simulink model "Sim_2025_04_07_Heet"  (R2024b)
settings: Solver=FixedStepAuto  StartTime=0.0  StopTime=2350  FixedStep=0.01  RelTol=1e-3
values from neighbouring files (symbols this model uses):
  cpSn = 230    [Sim_Parameter_Heet.m]
  mB = VB*rohSn    (= 7671.14496)    [Sim_Parameter_Heet.m]
  TU = 35    [Sim_Parameter_Heet.m]
undefined symbols (not defined in the file or in its folder): PLC_1, SIMATIC, UA
libraries: simulink x7, slpidlib x7, opcualib x6
(part 1 of 3)
settings Model: Creator=hartmann  LastModifiedBy=khamar

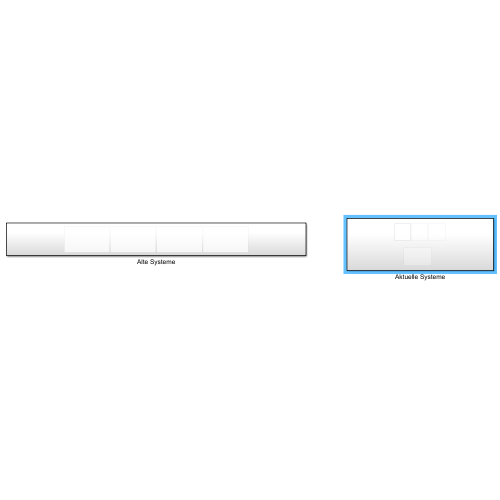
[thumbnail: Simulink's stored preview of the top-level diagram]
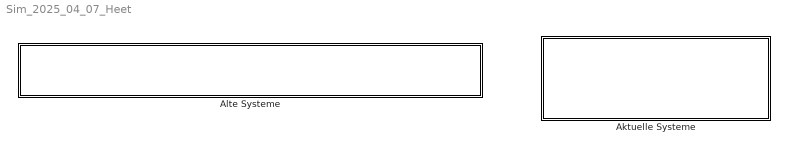
== system Sim_2025_04_07_Heet ==
  Aktuelle Systeme : Subsystem
  Alte Systeme : Subsystem

== system Sim_2025_04_07_Heet/Aktuelle Systeme ==
  Subsystem : Subsystem  Commented=on
  System für Stillstand für Siemens : Subsystem  Commented=on
  System mit Echtdatensätze : Subsystem
  System ohne Echtdatensätze : Subsystem  Commented=on

== system Sim_2025_04_07_Heet/Alte Systeme ==
  Subsystem1 : Subsystem  Commented=on
  Subsystem2 : Subsystem  Commented=on
  Subsystem3 : Subsystem  Commented=on
  Subsystem4 : Subsystem  Commented=on

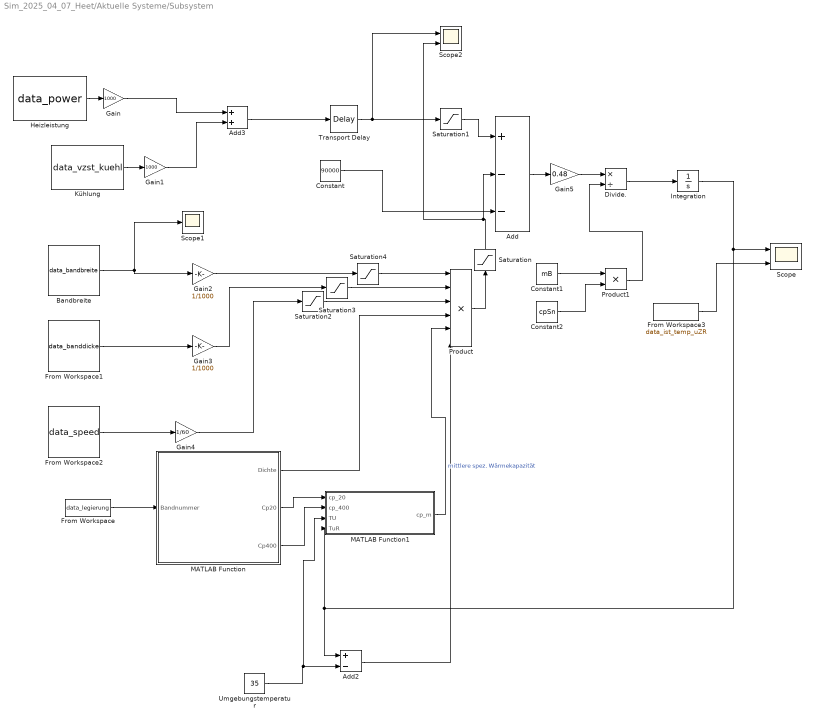
== system Sim_2025_04_07_Heet/Aktuelle Systeme/Subsystem ==
  Add : Sum  Inputs=+--
  Add2 : Sum  Inputs=+-
  Add3 : Sum
  Bandbreite : FromWorkspace  VariableName=data_bandbreite
  Constant : Constant  Value=90000
  Constant1 : Constant  Value=mB
  Constant2 : Constant  Value=cpSn
  Divide. : Product  Inputs=*/
  From Workspace : FromWorkspace  VariableName=data_legierung
  From Workspace1 : FromWorkspace  VariableName=data_banddicke
  From Workspace2 : FromWorkspace  VariableName=data_speed
  From Workspace3 : FromWorkspace  VariableName=data_ist_temp_uZR
  Gain : Gain  Gain=1000
  Gain1 : Gain  Gain=1000
  Gain2 : Gain  Gain=1/1000
  Gain3 : Gain  Gain=1/1000
  Gain4 : Gain  Gain=1/60
  Gain5 : Gain  Gain=0.48
  Heizleistung : FromWorkspace  VariableName=data_power
  Integration : Integrator  InitialCondition=273  IgnoreLimit=on
  Kühlung : FromWorkspace  VariableName=data_vzst_kuehl
  MATLAB Function : MATLAB Function  TreatAsAtomicUnit=on
  MATLAB Function1 : MATLAB Function  TreatAsAtomicUnit=on
  Product : Product  Inputs=6
  Product1 : Product
  Saturation{,1..4} (5 alike) : Saturate  UpperLimit=inf  LowerLimit=0
  Scope : Scope  NumInputPorts=2
  Scope1 : Scope
  Scope2 : Scope  NumInputPorts=2
  Transport Delay : TransportDelay  DelayTime=95
  Umgebungstemperatur : Constant  Value=35
  wires:
  Heizleistung/1 -> Gain/1
  Kühlung/1 -> Gain1/1
  Add3/1 -> Transport Delay/1
  Bandbreite/1 -> Scope1/1, Gain2/1
  From Workspace1/1 -> Gain3/1
  From Workspace2/1 -> Gain4/1
  Product/1 -> Saturation/1
  Divide./1 -> Integration/1
  Integration/1 -> Add2/1, MATLAB Function1/4(TuR), Scope/1
  Add/1 -> Gain5/1
  From Workspace/1 -> MATLAB Function/1(Bandnummer)
  MATLAB Function/1(Dichte) -> Product/4
  MATLAB Function/2(Cp20) -> MATLAB Function1/1(cp_20)
  MATLAB Function/3(Cp400) -> MATLAB Function1/2(cp_400)
  Constant1/1 -> Product1/1
  Constant2/1 -> Product1/2
  Product1/1 -> Divide./2
  Umgebungstemperatur/1 -> MATLAB Function1/3(TU), Add2/2
  Add2/1 -> Product/6
  From Workspace3/1 -> Scope/2
  Saturation/1 -> Scope2/2, Add/2
  Saturation1/1 -> Add/1
  Gain/1 -> Add3/1
  Gain1/1 -> Add3/2
  Gain2/1 -> Saturation4/1
  Gain3/1 -> Saturation3/1
  Gain4/1 -> Saturation2/1
  MATLAB Function1/1(cp_m) -> Product/5  "mittlere spez. Wärmekapazität"
  Constant/1 -> Add/3
  Saturation2/1 -> Product/3
  Saturation3/1 -> Product/2
  Saturation4/1 -> Product/1
  Gain5/1 -> Divide./1
  Transport Delay/1 -> Scope2/1, Saturation1/1

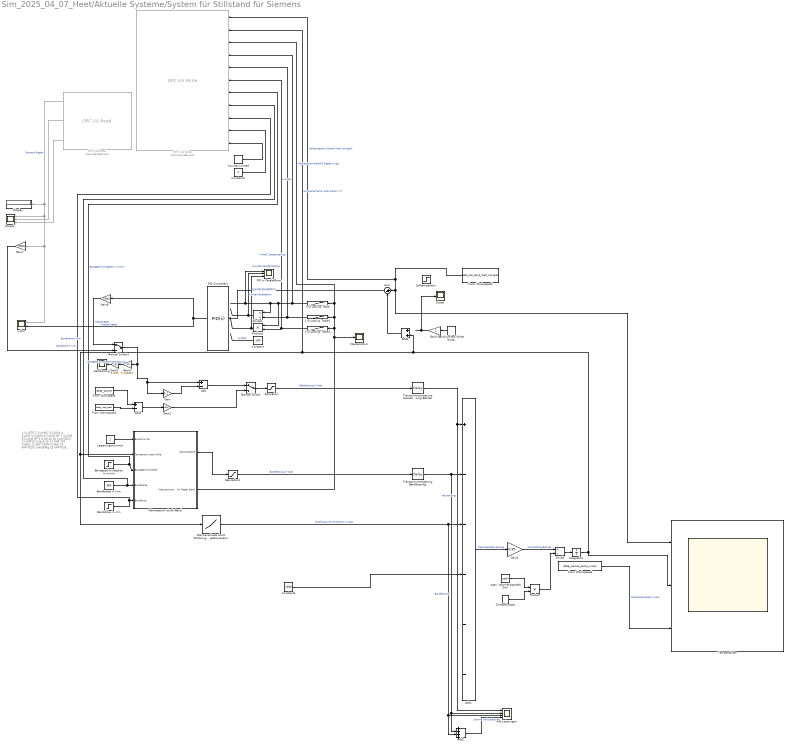
== system Sim_2025_04_07_Heet/Aktuelle Systeme/System für Stillstand für Siemens ==
  note: 1
      | Cu-ETP
      |
      | 2
      | Cu-PHC
      |
      | 3
      | CuSn4
      |
      | 4
      | CuSn5
      |
      | 5
      | CuSn6
      |
      | 6
      | CuSn6 HP
      |
      | 7
      | CuSn8
      |
      | 8
      | CuSn8 HP
      |
      | 9
      | CuSn10
      |
      | 10
      | CuSn3Zn9
      |
      | 11
      | KHP15 CuSn0,15
      |
      | 12
      | KHP 102 CuNiSi
      |
      | 13
      | KHP 102M CuNiSi
      |
      | 14
      | KHP7025 CuNi3SiMg
      |
      | 15
      | KHP7026 CuNi2Si
      |
      | 16
      | KHP105 CuNi1Sn0,5
      |
      | 17
      | KHP109 CuNi1Sn0,9
      |
      | 18
      | C688 CuZn23Al3,5Co
  1-D Lookup Table : Lookup_n-D  NumberOfTableDimensions=1  BreakpointsForDimension1=[0 0.10000000000000001 0.20000000000000001 0.29999999999999999 0.40000000000000002 0.5 0.59999999999999998 0.69999999999999996 0.80000000000000004 0.90000000000000002 1 1.1000000000000001 1.2 1.3 1.3999999999999999 1.5 1.6000000000000001 1.7 1.8 1.8999999999999999 2 2.1000000000000001 2.2000000000000002 2.2999999999999998 2.3999999999999999 2.5 2.6000000000000001 2.7000000000000002 2.7999999999999998 2.8999999999999999 3 3.1000000000000001 3.2000000000000002 3.2999999999999998 3.3999999999999999 3.5 3.6000000000000001 3.7000000000000002 3.7999999999999998 3.8999999999999999 4 4.0999999999999996 4.2000000000000002 4.2999999999999998 4.4000000000000004 4.5]  Table=[5;5.07;5.13;5.2;5.27;5.33;5.4;5.47;5.53;5.6;5.67;5.73;5.8;5.87;5.93;6;6.07;6.13;6.2;6.27;6.33;6.4;6.47;6.53;6.6;6.67;6.73;6.8;6.87;6.93;7;7.07;7.13;7.2;7.27;7.33;7.4;7.47;7.53;7.6;7.67;7.73;7.8;7.87;7.93;8]  InternalRulePriority=Speed  RndMeth=Simplest
  1-D Lookup Table1 : Lookup_n-D  NumberOfTableDimensions=1  BreakpointsForDimension1=[0 0.10000000000000001 0.20000000000000001 0.29999999999999999 0.40000000000000002 0.5 0.59999999999999998 0.69999999999999996 0.80000000000000004 0.90000000000000002 1 1.1000000000000001 1.2 1.3 1.3999999999999999 1.5 1.6000000000000001 1.7 1.8 1.8999999999999999 2 2.1000000000000001 2.2000000000000002 2.2999999999999998 2.3999999999999999 2.5 2.6000000000000001 2.7000000000000002 2.7999999999999998 2.8999999999999999 3 3.1000000000000001 3.2000000000000002 3.2999999999999998 3.3999999999999999 3.5 3.6000000000000001 3.7000000000000002 3.7999999999999998 3.8999999999999999 4 4.0999999999999996 4.2000000000000002 4.2999999999999998 4.4000000000000004 4.5]  Table=[285.7;253.3;256.7;260;263.3;266.7;270;273.3;276.7;280;283.3;286.7;290;293.3;296.7;300;303.3;306.7;310;313.3;316.7;320;323.3;326.7;330;333.3;336.7;340;343.3;346.7;350;353.3;356.7;360;363.3;366.7;370;373.3;376.7;380;383.3;386.7;390;393.3;396.7;400]  InternalRulePriority=Speed  RndMeth=Simplest
  1-D Lookup Table2 : Lookup_n-D  NumberOfTableDimensions=1  BreakpointsForDimension1=[0 0.10000000000000001 0.20000000000000001 0.29999999999999999 0.40000000000000002 0.5 0.59999999999999998 0.69999999999999996 0.80000000000000004 0.90000000000000002 1 1.1000000000000001 1.2 1.3 1.3999999999999999 1.5 1.6000000000000001 1.7 1.8 1.8999999999999999 2 2.1000000000000001 2.2000000000000002 2.2999999999999998 2.3999999999999999 2.5 2.6000000000000001 2.7000000000000002 2.7999999999999998 2.8999999999999999 3 3.1000000000000001 3.2000000000000002 3.2999999999999998 3.3999999999999999 3.5 3.6000000000000001 3.7000000000000002 3.7999999999999998 3.8999999999999999 4 4.0999999999999996 4.2000000000000002 4.2999999999999998 4.4000000000000004 4.5]  Table=[8;59.2;58.4;57.7;57;56.3;55.6;54.9;54.2;53.6;52.9;52.3;51.7;51.1;50.6;50;49.5;48.9;48.4;47.9;47.4;46.9;46.4;45.9;45.5;45;44.6;44.1;43.7;43.3;42.9;42.5;42.1;41.7;41.3;40.9;40.5;40.2;39.8;39.5;39.1;38.8;38.5;38.1;37.8;37.5]  InternalRulePriority=Speed  RndMeth=Simplest
  Add : Sum  Inputs=+-
  Add1 : Sum  Inputs=+-----
  Add2 : Sum  Inputs=++++
  Add3 : Sum
  Add4 : Sum  Inputs=+-
  Alle Leistungen : Scope  NumInputPorts=6
  Band-Limited White Noise : simulink/Sources/Band-Limited White Noise  Cov=[0.1]  Ts=20  seed=[23341]
  Bandbreite in mm : Constant  Value=360
  Banddicke in mm : Step  Time=3000  Before=0.15  After=0.5  SampleTime=0
  Bandgeschwindigkeit in m/min : Step  Time=2000  After=0  SampleTime=0
  Constant : Constant  Value=100
  Constant1 : Constant  Value=-1000
  Constant2 : Constant
  Counter Limited : simulink/Sources/Counter Limited  uplimit=100  tsamp=-1
  Display : Display
  Divide : Product  Inputs=*/
  Divide1 : Product  Inputs=*/
  From Workspace : FromWorkspace  VariableName=data_power
  From Workspace1 : FromWorkspace  VariableName=data_vzst_kuehl
  From Workspace2 : FromWorkspace  VariableName=data_soll_temp_start_korrigiert
  From Workspace3 : FromWorkspace  VariableName=data_wanne_temp_innen
  Gain : Gain  Gain=0.1
  Gain1 : Gain
  Gain2 : Gain  Gain=1000
  Gain3 : Gain  Gain=0.95
  Gain4 : Gain  Gain=0.142857
  Gain5 : Gain  Gain=0.001
  Gain7 : Gain  Gain=7000
  Gain9 : Gain  Gain=7000
  Heizleistung : Scope
  Integration : Integrator  InitialCondition=276.5  IgnoreLimit=on
  Legierungsnummer : Constant
  Manual Switch : ManualSwitch
  Manual Switch1 : ManualSwitch
  Massenstrom : Scope
  OPC UA Read : opcualib/OPC UA Read  Commented=on  SelectedServer=SIMATIC.S7-1500.OPC-UA.Application:PLC_1  ServerList=SIMATIC.S7-1500.OPC-UA.Application:PLC_1  NodeList={ '1', 'reStellwert', '4', '2', '1' }  ShowQualityPort=on  ShowTimestampPort=on  ShowTimestampPortAs=Seconds since start  SampleTime=-1
  OPC UA Write : opcualib/OPC UA Write  Commented=on  SelectedServer=SIMATIC.S7-1500.OPC-UA.Application:PLC_1  ServerList=SIMATIC.S7-1500.OPC-UA.Application:PLC_1  SampleTime=-1  NodeList={ '1', 'reSollwert', '4', '3', '1'; '2', 'reIstTemperaturVonStreckensimulation', '4', '4', '1'; '3', 'reMassenfluss', '4', '5', '1'; '4', 'reP_Anteil', '4', '6', '1'; '5', 'reI_Anteil', '4', '7', '1'; '6', 'reD_Anteil', '4', '8', '1'; '7', 'reGeschwindigkeit', '4', '9', '1'; '8', 'reBandbreite', '4', '10', '1'; '9', 'reBanddicke', '4', '11', '1'; '10', 'boRunVonSimulink', '4', '12', '1'; '11', 'iLifeRegister', '4', '13', '1' }
  PID Controller1 : slpidlib/PID Controller  Controller=PID  Form=Parallel  TimeDomain=Continuous-time  UseExternalTs=off  SampleTime=-1  IntegratorMethod=Forward Euler  FilterMethod=Forward Euler  ControllerParametersSource=internal  P=5  I=0.0175  UseKiTs=off  D=40  UseExternalDerivativeSource=off  N=1  UseFilter=on  TunerSelectOption=Transfer Function Based (PID Tuner App)  InitialConditionSource=internal  InitialConditionForIntegrator=0  InitialConditionForFilter=0  DifferentiatorICPrevScaledInput=0  ExternalReset=none  TrackingMode=off  Kt=1  LimitOutput=on  SatLimitsSource=internal  UpperSaturationLimit=100  LowerSaturationLimit=0  LinearizeAsGain=on  AntiWindupMode=none  Kb=1  LimitIntegrator=off  UpperIntegratorSaturationLimit=inf  LowerIntegratorSaturationLimit=-inf  POutMin=[]  POutMax=[]  IOutMin=[]  IOutMax=[]  DOutMin=[]  DOutMax=[]  NOutMin=[]  NOutMax=[]  SumOutMin=[]  SumOutMax=[]  SaturationOutMin=[]  SaturationOutMax=[]  PParamMin=[]  PParamMax=[]  IParamMin=[]  IParamMax=[]  DParamMin=[]  DParamMax=[]  NParamMin=[]  NParamMax=[]  KbParamMin=[]  KbParamMax=[]  KtParamMin=[]  KtParamMax=[]  KbOutMin=[]  KbOutMax=[]  KtOutMin=[]  KtOutMax=[]  IntegratorOutMin=[]  IntegratorOutMax=[]  FilterOutMin=[]  FilterOutMax=[]  SumI1OutMin=[]  SumI1OutMax=[]  SumI2OutMin=[]  SumI2OutMax=[]  SumI3OutMin=[]  SumI3OutMax=[]  SumI4OutMin=[]  SumI4OutMax=[]  SumDOutMin=[]  SumDOutMax=[]  DifferentiatorOutMin=[]  DifferentiatorOutMax=[]  FilterDiffOutCoefMin=[]  FilterDiffOutCoefMax=[]  ReciprocalOutMin=[]  ReciprocalOutMax=[]  SumDenOutMin=[]  SumDenOutMax=[]  SumNumOutMin=[]  SumNumOutMax=[]  DivideOutMin=[]  DivideOutMax=[]  UdiffTsProdOutMin=[]  UdiffTsProdOutMax=[]  NTsProdOutMin=[]  NTsProdOutMax=[]  UintegralTsProdOutMin=[]  UintegralTsProdOutMax=[]  UngainTsProdOutMin=[]  UngainTsProdOutMax=[]  ClampingZeroOutDataTypeStr=Inherit: Inherit via back propagation  ClampingZeroOutMin=[]  ClampingZeroOutMax=[]  FilterDenConstantOutDataTypeStr=Inherit: Inherit via back propagation  FilterDenConstantOutMin=[]  FilterDenConstantOutMax=[]  PCopyOutDataTypeStr=Inherit: Inherit via back propagation  PCopyOutMin=[]  PCopyOutMax=[]  NCopyOutDataTypeStr=Inherit: Inherit via back propagation  NCopyOutMin=[]  NCopyOutMax=[]  IntegratorContinuousStateAttributes=''  IntegratorStateMustResolveToSignalObject=off  IntegratorRTWStateStorageClass=Auto  FilterContinuousStateAttributes=''  FilterStateMustResolveToSignalObject=off  FilterRTWStateStorageClass=Auto  ParallelPVariant=InternalParameters  IdealPVariant=Disabled  IVariant=InternalParameters  DVariant=InternalParameters  IntegratorVariant=Continuous  SatVariant=Enabled  AWVariant=Passthrough  PCopyVariant=Disabled  TRVariant=Disabled  FdbkBlocksVariant=Forward  IdealPFdbkVariant=Disabled  SatFdbkVariant=Disabled  DerivativeFilterVariant=ContFilter  NVariant=InternalParameters  NCopyVariant=Disabled  FilterICVariant=InternalICsFilter  IntegratorICVariant=InternalICs  ExternalResetVariant=Disabled  TRSumVariant=Passthrough  SumFdbkVariant=Disabled  SumVariant=Sum_PID  TsampFilterVariant=InternalTs  TsampNgainVariant=Passthrough  TsampIntegralVariant=Disabled_SignalSpec  ExternalSaturationOutDataTypeStr=Inherit: Same as second input  DerivativeSourceVariant=ErrorSignal  PreIntVariant=InternalPreInt
  PID in Paralellform : Scope  NumInputPorts=3
  Product : Product
  Product1 : Product
  Saturation : Saturate  UpperLimit=inf  LowerLimit=0
  Saturation1 : Saturate  UpperLimit=inf  LowerLimit=0
  Scope : Scope
  Scope1 : Scope  NumInputPorts=3
  Solltemperatur : Step  Time=1000  Before=277  After=279  SampleTime=0
  Sum : Sum  Inputs=|+-
  Temperaturen : Scope  NumInputPorts=3
  Transportverzögerung Bandleistung : TransportDelay  DelayTime=5
  Transportverzögerung Heizleistung Betrieb : TransportDelay  DelayTime=63  BufferSize=15000
  Wärmestrom durch Band : Subsystem
  "Wärmeverluste durch Strahlung und Konvektion in Abhängigkeit der Zinntemperatur, mit fester Umgebungstemperatur" : Lookup_n-D  NumberOfTableDimensions=1  BreakpointsForDimension1=[0 250 260 270 280 290 300 310 320]  Table=[0;15000;15200;15400;15600;15800;16000;16200;16400]  InternalRulePriority=Speed  RndMeth=Simplest
  Zinnbadmasse : Constant  Value=7700
  spez. Wärmekapazität Zinn : Constant  Value=cpSn
  y-Out : Scope  NumInputPorts=2
  wires:
  Product/1 -> Divide/2
  Saturation1/1 -> Transportverzögerung Bandleistung/1  "Bandleistung in Watt"
  PID Controller1/1 -> Gain9/1, y-Out/2  "Matlab-Regler"
  Transportverzögerung Bandleistung/1 -> Alle Leistungen/3, Add2/2, Add1/2  "Bandleistung"
  Banddicke in mm/1 -> OPC UA Write/9, Wärmestrom durch Band/5(Banddicke)  "Banddicke in mm"
  Legierungsnummer/1 -> Wärmestrom durch Band/1(Bandnummer)
  Saturation/1 -> Transportverzögerung Heizleistung Betrieb/1  "Ofenleistung in Watt"
  Gain5/1 -> Heizleistung/1  "Geregelte simulierte Heizleistung"
  Bandgeschwindigkeit in m/min/1 -> OPC UA Write/7, Wärmestrom durch Band/3(Bandgeschwindikeit)  "Bandgeschwindigkeit in m/min"
  Gain4/1 -> Gain5/1
  spez. Wärmekapazität Zinn/1 -> Product/1
  Divide/1 -> Integration/1
  Sum/1 -> PID Controller1/1
  Integration/1 -> OPC UA Write/2, Wärmestrom durch Band/2(Temperatur unter Rolle), "Wärmeverluste durch Strahlung und Konvektion in Abhängigkeit der Zinntemperatur, mit fester Umgebungstemperatur"/1, Add3/2, Temperaturen/2  "Simulierte Temp. unter Rolle in °C"
  Zinnbadmasse/1 -> Product/2
  "Wärmeverluste durch Strahlung und Konvektion in Abhängigkeit der Zinntemperatur, mit fester Umgebungstemperatur"/1 -> Alle Leistungen/4, Add2/3, Add1/3  "Strahlung und Konvektion in Watt"
  Gain3/1 -> Divide/1  "Wirkleistung Betrieb"
  Wärmestrom durch Band/1(Leistung Band) -> Saturation1/1
  Constant/1 -> ?  "N-Filter"
  Wärmestrom durch Band/2(Massenstrom für Regler Band) -> Massenstrom/1, OPC UA Write/3, 1-D Lookup Table/1, 1-D Lookup Table1/1, 1-D Lookup Table2/1  "Massenstrom Band für Regler in kg/s"
  From Workspace2/1 -> OPC UA Write/1, Temperaturen/1, Sum/1  "Solltemperatur Wanne innen korrigiert"
  Transportverzögerung Heizleistung Betrieb/1 -> Alle Leistungen/1, Add1/1  "Heizleistung"
  Add/1 -> Manual Switch/1
  OPC UA Read/2 -> Scope1/2
  OPC UA Read/1 -> Display/1, Scope1/1, Gain7/1, y-Out/1  "Siemens-Regler"
  OPC UA Read/3 -> Scope1/3
  Add2/1 -> Alle Leistungen/6  "Summe Verlustleistung"
  Add1/1 -> Gain3/1  "Resultierende Leistung"
  Constant2/1 -> OPC UA Write/10
  Counter Limited/1 -> OPC UA Write/11
  Gain7/1 -> Manual Switch1/2
  Gain9/1 -> Manual Switch1/1  "Matlabregler"
  1-D Lookup Table/1 -> Product1/1, Divide1/1, PID in Paralellform/1, OPC UA Write/4  "P-Anteil"
  1-D Lookup Table1/1 -> OPC UA Write/5, Divide1/2  "I-Anteil Zeitdarstellung"
  1-D Lookup Table2/1 -> Product1/2, OPC UA Write/6  "D-Anteil Zeitdarstellung"
  Bandbreite in mm/1 -> OPC UA Write/8, Wärmestrom durch Band/4(Bandbreite)  "Bandbreite in mm"
  Divide1/1 -> PID in Paralellform/2  "I-Anteil Parallelform"
  Product1/1 -> PID in Paralellform/3  "D-Anteil Paralellform"
  Gain/1 -> Add/2
  Band-Limited White Noise/1 -> Gain1/1
  Add3/1 -> Sum/2
  Gain1/1 -> Scope/1
  From Workspace/1 -> Add4/1
  Manual Switch1/1 -> Gain/1, Add/1, Gain4/1
  From Workspace1/1 -> Add4/2
  Add4/1 -> Gain2/1
  Manual Switch/1 -> Saturation/1
  Gain2/1 -> Manual Switch/2
  Constant1/1 -> Add1/4
  From Workspace3/1 -> Temperaturen/3  "Wannentemperatur innen"
  ? -> ?  "Temperatur unter Rolle"
  ? -> ?  "Soll-Temp. unter Rolle"
  ? -> ?  "Wannentemperatur außen"
  ? -> ?  "Solltemperatur Wanne innen Rezept"

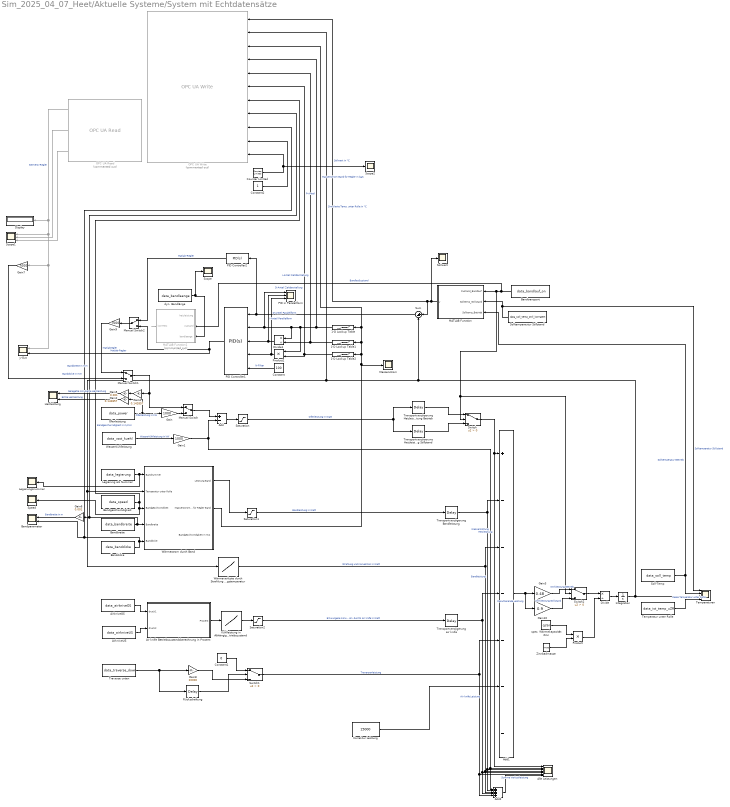
== system Sim_2025_04_07_Heet/Aktuelle Systeme/System mit Echtdatensätze ==
  1-D Lookup Table : Lookup_n-D  NumberOfTableDimensions=1  BreakpointsForDimension1=[0 0.29999999999999999 0.59999999999999998 0.90000000000000002 1.2 1.5 1.8 2.1000000000000001 2.3999999999999999 2.7000000000000002 3 3.2999999999999998 3.6000000000000001 3.8999999999999999 4.2000000000000002 4.5]  Table=[5;5.2;5.4;5.6;5.8;6;6.2;6.4;6.6;6.8;7;7.2;7.4;7.6;7.8;8]  InternalRulePriority=Speed  RndMeth=Simplest
  1-D Lookup Table1 : Lookup_n-D  NumberOfTableDimensions=1  BreakpointsForDimension1=[0 0.29999999999999999 0.59999999999999998 0.90000000000000002 1.2 1.5 1.8 2.1000000000000001 2.3999999999999999 2.7000000000000002 3 3.2999999999999998 3.6000000000000001 3.8999999999999999 4.2000000000000002 4.5]  Table=[250;260;270;280;290;300;310;320;330;340;350;360;370;380;390;400]  InternalRulePriority=Speed  RndMeth=Simplest
  1-D Lookup Table2 : Lookup_n-D  NumberOfTableDimensions=1  BreakpointsForDimension1=[0 0.29999999999999999 0.59999999999999998 0.90000000000000002 1.2 1.5 1.8 2.1000000000000001 2.3999999999999999 2.7000000000000002 3 3.2999999999999998 3.6000000000000001 3.8999999999999999 4.2000000000000002 4.5]  Table=[60;57.7;55.6;53.6;51.7;50;48.4;46.9;45.5;44.1;42.9;41.7;40.5;39.5;38.5;37.5]  InternalRulePriority=Speed  RndMeth=Simplest
  Add : Sum  Inputs=+-
  Add1 : Sum  Inputs=+------
  Add2 : Sum  Inputs=+++++
  Air knife Betriebszustandsberechnung in Prozent : MATLAB Function  TreatAsAtomicUnit=on  SystemSampleTime=0.1
  AirkniveOS : FromWorkspace  VariableName=data_airkniveOS  SampleTime=-1
  AirkniveUS : FromWorkspace  VariableName=data_airkniveUS  SampleTime=-1
  Alle Leistungen : Scope  NumInputPorts=7
  Bandbreite : FromWorkspace  VariableName=data_bandbreite  SampleTime=-1
  Banddicke : FromWorkspace  VariableName=data_banddicke  SampleTime=-1
  Bandgeschwindigkeit : FromWorkspace  VariableName=data_speed  SampleTime=-1
  Bandparameter : Scope  NumInputPorts=2
  Bandtransport : FromWorkspace  VariableName=data_bandlauf_on  SampleTime=-1
  Constant : Constant  Value=100
  Constant1 : Constant  Value=0
  Constant2 : Constant
  Counter Limited : simulink/Sources/Counter Limited  uplimit=100  tsamp=-1
  Display : Display
  Divide : Product  Inputs=*/
  Divide1 : Product  Inputs=*/  OutMin=[eps]
  Gain : Gain  Gain=1000
  Gain1 : Gain  Gain=1000
  Gain10 : Gain  Gain=0.9
  Gain2 : Gain  Gain=0.142857
  Gain3 : Gain  Gain=0.48
  Gain4 : Gain  Gain=0.142857
  Gain5 : Gain  Gain=0.001
  Gain6 : Gain  Gain=0.001
  Gain7 : Gain  Gain=7000
  Gain8 : Gain  Gain=20000
  Gain9 : Gain  Gain=7000
  Heizleistung : Scope  NumInputPorts=2
  Integration : Integrator  InitialCondition=275  IgnoreLimit=on
  Korrektur Leistung : Constant  Value=15000
  Kühlleistung in Abhängigkeit des Betriebszustand : Lookup_n-D  NumberOfTableDimensions=1  BreakpointsForDimension1=[0 50 70 80 90 100]  Table=[0 17000 19500 19700 19900 19800]  InternalRulePriority=Speed  RndMeth=Simplest
  Legierung als Nummer : FromWorkspace  VariableName=data_legierung
  Legierungsnummer : Scope
  MATLAB Function : MATLAB Function  TreatAsAtomicUnit=on
  MATLAB Function1 : MATLAB Function  Commented=on  TreatAsAtomicUnit=on
  Manual Switch : ManualSwitch
  Manual Switch1 : ManualSwitch
  Manual Switch2 : ManualSwitch
  Massenstrom : Scope
  OPC UA Read : opcualib/OPC UA Read  Commented=on  SelectedServer=SIMATIC.S7-1500.OPC-UA.Application:PLC_1  ServerList=SIMATIC.S7-1500.OPC-UA.Application:PLC_1  NodeList={ '1', 'reStellwert', '4', '2', '1' }  ShowQualityPort=on  ShowTimestampPort=on  ShowTimestampPortAs=Seconds since start  SampleTime=-1
  OPC UA Write : opcualib/OPC UA Write  Commented=on  SelectedServer=SIMATIC.S7-1500.OPC-UA.Application:PLC_1  ServerList=SIMATIC.S7-1500.OPC-UA.Application:PLC_1  SampleTime=-1  NodeList={ '1', 'reSollwert', '4', '3', '1'; '2', 'reIstTemperaturVonStreckensimulation', '4', '4', '1'; '3', 'reMassenfluss', '4', '5', '1'; '4', 'reP_Anteil', '4', '6', '1'; '5', 'reI_Anteil', '4', '7', '1'; '6', 'reD_Anteil', '4', '8', '1'; '7', 'reGeschwindigkeit', '4', '9', '1'; '8', 'reBandbreite', '4', '10', '1'; '9', 'reBanddicke', '4', '11', '1'; '10', 'boRunVonSimulink', '4', '12', '1'; '11', 'iLifeRegister', '4', '13', '1' }
  Ofenleistung : FromWorkspace  VariableName=data_power  SampleTime=-1  OutputAfterFinalValue=Setting to zero
  PID Controller1 : slpidlib/PID Controller  Controller=PID  Form=Parallel  TimeDomain=Continuous-time  UseExternalTs=off  SampleTime=-1  IntegratorMethod=Forward Euler  FilterMethod=Forward Euler  ControllerParametersSource=external  P=4.4  I=0.02  UseKiTs=off  D=29.92  UseExternalDerivativeSource=off  N=1  UseFilter=on  TunerSelectOption=Transfer Function Based (PID Tuner App)  InitialConditionSource=internal  InitialConditionForIntegrator=0  InitialConditionForFilter=0  DifferentiatorICPrevScaledInput=0  ExternalReset=none  TrackingMode=off  Kt=1  LimitOutput=on  SatLimitsSource=internal  UpperSaturationLimit=100  LowerSaturationLimit=0  LinearizeAsGain=on  AntiWindupMode=none  Kb=1  LimitIntegrator=off  UpperIntegratorSaturationLimit=inf  LowerIntegratorSaturationLimit=-inf  POutMin=[]  POutMax=[]  IOutMin=[]  IOutMax=[]  DOutMin=[]  DOutMax=[]  NOutMin=[]  NOutMax=[]  SumOutMin=[]  SumOutMax=[]  SaturationOutMin=[]  SaturationOutMax=[]  PParamMin=[]  PParamMax=[]  IParamMin=[]  IParamMax=[]  DParamMin=[]  DParamMax=[]  NParamMin=[]  NParamMax=[]  KbParamMin=[]  KbParamMax=[]  KtParamMin=[]  KtParamMax=[]  KbOutMin=[]  KbOutMax=[]  KtOutMin=[]  KtOutMax=[]  IntegratorOutMin=[]  IntegratorOutMax=[]  FilterOutMin=[]  FilterOutMax=[]  SumI1OutMin=[]  SumI1OutMax=[]  SumI2OutMin=[]  SumI2OutMax=[]  SumI3OutMin=[]  SumI3OutMax=[]  SumI4OutMin=[]  SumI4OutMax=[]  SumDOutMin=[]  SumDOutMax=[]  DifferentiatorOutMin=[]  DifferentiatorOutMax=[]  FilterDiffOutCoefMin=[]  FilterDiffOutCoefMax=[]  ReciprocalOutMin=[]  ReciprocalOutMax=[]  SumDenOutMin=[]  SumDenOutMax=[]  SumNumOutMin=[]  SumNumOutMax=[]  DivideOutMin=[]  DivideOutMax=[]  UdiffTsProdOutMin=[]  UdiffTsProdOutMax=[]  NTsProdOutMin=[]  NTsProdOutMax=[]  UintegralTsProdOutMin=[]  UintegralTsProdOutMax=[]  UngainTsProdOutMin=[]  UngainTsProdOutMax=[]  ClampingZeroOutDataTypeStr=Inherit: Inherit via back propagation  ClampingZeroOutMin=[]  ClampingZeroOutMax=[]  FilterDenConstantOutDataTypeStr=Inherit: Inherit via back propagation  FilterDenConstantOutMin=[]  FilterDenConstantOutMax=[]  PCopyOutDataTypeStr=Inherit: Inherit via back propagation  PCopyOutMin=[]  PCopyOutMax=[]  NCopyOutDataTypeStr=Inherit: Inherit via back propagation  NCopyOutMin=[]  NCopyOutMax=[]  IntegratorContinuousStateAttributes=''  IntegratorStateMustResolveToSignalObject=off  IntegratorRTWStateStorageClass=Auto  FilterContinuousStateAttributes=''  FilterStateMustResolveToSignalObject=off  FilterRTWStateStorageClass=Auto  ParallelPVariant=ExternalParameters  IdealPVariant=Disabled  IVariant=ExternalParameters  DVariant=ExternalParameters  IntegratorVariant=Continuous  SatVariant=Enabled  AWVariant=Passthrough  PCopyVariant=Disabled  TRVariant=Disabled  FdbkBlocksVariant=Forward  IdealPFdbkVariant=Disabled  SatFdbkVariant=Disabled  DerivativeFilterVariant=ContFilter  NVariant=ExternalParameters  NCopyVariant=Disabled  FilterICVariant=InternalICsFilter  IntegratorICVariant=InternalICs  ExternalResetVariant=Disabled  TRSumVariant=Passthrough  SumFdbkVariant=Disabled  SumVariant=Sum_PID  TsampFilterVariant=InternalTs  TsampNgainVariant=Passthrough  TsampIntegralVariant=Disabled_SignalSpec  ExternalSaturationOutDataTypeStr=Inherit: Same as second input  DerivativeSourceVariant=ErrorSignal  PreIntVariant=InternalPreInt
  PID Controller2 : slpidlib/PID Controller  Controller=PID  Form=Parallel  TimeDomain=Continuous-time  UseExternalTs=off  SampleTime=-1  IntegratorMethod=Forward Euler  FilterMethod=Forward Euler  ControllerParametersSource=internal  P=7  I=0.04  UseKiTs=off  D=300  UseExternalDerivativeSource=off  N=1  UseFilter=on  TunerSelectOption=Transfer Function Based (PID Tuner App)  InitialConditionSource=internal  InitialConditionForIntegrator=0  InitialConditionForFilter=0  DifferentiatorICPrevScaledInput=0  ExternalReset=none  TrackingMode=off  Kt=1  LimitOutput=on  SatLimitsSource=internal  UpperSaturationLimit=100  LowerSaturationLimit=0  LinearizeAsGain=on  AntiWindupMode=none  Kb=1  LimitIntegrator=off  UpperIntegratorSaturationLimit=inf  LowerIntegratorSaturationLimit=-inf  POutMin=[]  POutMax=[]  IOutMin=[]  IOutMax=[]  DOutMin=[]  DOutMax=[]  NOutMin=[]  NOutMax=[]  SumOutMin=[]  SumOutMax=[]  SaturationOutMin=[]  SaturationOutMax=[]  PParamMin=[]  PParamMax=[]  IParamMin=[]  IParamMax=[]  DParamMin=[]  DParamMax=[]  NParamMin=[]  NParamMax=[]  KbParamMin=[]  KbParamMax=[]  KtParamMin=[]  KtParamMax=[]  KbOutMin=[]  KbOutMax=[]  KtOutMin=[]  KtOutMax=[]  IntegratorOutMin=[]  IntegratorOutMax=[]  FilterOutMin=[]  FilterOutMax=[]  SumI1OutMin=[]  SumI1OutMax=[]  SumI2OutMin=[]  SumI2OutMax=[]  SumI3OutMin=[]  SumI3OutMax=[]  SumI4OutMin=[]  SumI4OutMax=[]  SumDOutMin=[]  SumDOutMax=[]  DifferentiatorOutMin=[]  DifferentiatorOutMax=[]  FilterDiffOutCoefMin=[]  FilterDiffOutCoefMax=[]  ReciprocalOutMin=[]  ReciprocalOutMax=[]  SumDenOutMin=[]  SumDenOutMax=[]  SumNumOutMin=[]  SumNumOutMax=[]  DivideOutMin=[]  DivideOutMax=[]  UdiffTsProdOutMin=[]  UdiffTsProdOutMax=[]  NTsProdOutMin=[]  NTsProdOutMax=[]  UintegralTsProdOutMin=[]  UintegralTsProdOutMax=[]  UngainTsProdOutMin=[]  UngainTsProdOutMax=[]  ClampingZeroOutDataTypeStr=Inherit: Inherit via back propagation  ClampingZeroOutMin=[]  ClampingZeroOutMax=[]  FilterDenConstantOutDataTypeStr=Inherit: Inherit via back propagation  FilterDenConstantOutMin=[]  FilterDenConstantOutMax=[]  PCopyOutDataTypeStr=Inherit: Inherit via back propagation  PCopyOutMin=[]  PCopyOutMax=[]  NCopyOutDataTypeStr=Inherit: Inherit via back propagation  NCopyOutMin=[]  NCopyOutMax=[]  IntegratorContinuousStateAttributes=''  IntegratorStateMustResolveToSignalObject=off  IntegratorRTWStateStorageClass=Auto  FilterContinuousStateAttributes=''  FilterStateMustResolveToSignalObject=off  FilterRTWStateStorageClass=Auto  ParallelPVariant=InternalParameters  IdealPVariant=Disabled  IVariant=InternalParameters  DVariant=InternalParameters  IntegratorVariant=Continuous  SatVariant=Enabled  AWVariant=Passthrough  PCopyVariant=Disabled  TRVariant=Disabled  FdbkBlocksVariant=Forward  IdealPFdbkVariant=Disabled  SatFdbkVariant=Disabled  DerivativeFilterVariant=ContFilter  NVariant=InternalParameters  NCopyVariant=Disabled  FilterICVariant=InternalICsFilter  IntegratorICVariant=InternalICs  ExternalResetVariant=Disabled  TRSumVariant=Passthrough  SumFdbkVariant=Disabled  SumVariant=Sum_PID  TsampFilterVariant=InternalTs  TsampNgainVariant=Passthrough  TsampIntegralVariant=Disabled_SignalSpec  ExternalSaturationOutDataTypeStr=Inherit: Same as second input  DerivativeSourceVariant=ErrorSignal  PreIntVariant=InternalPreInt
  PID in Paralellform : Scope  NumInputPorts=3
  Product : Product
  Product1 : Product
  Rückschaltung : TransportDelay  DelayTime=20  BufferSize=20480
  Saturation : Saturate  UpperLimit=inf  LowerLimit=0
  Saturation1 : Saturate  UpperLimit=inf  LowerLimit=0
  Saturation2 : Saturate  UpperLimit=inf  LowerLimit=0
  Scope : Scope
  Scope1 : Scope  NumInputPorts=3
  Scope2 : Scope
  Soll-Temp : FromWorkspace  VariableName=data_soll_temp  SampleTime=-1
  Solltemperautur Stillstand : FromWorkspace  VariableName=data_soll_temp_still_korrigiert  SampleTime=-1
  Sollwert : Scope
  Speed : Scope
  Sum : Sum  Inputs=|+-
  Switch : Switch  Criteria=u2 > Threshold  SaturateOnIntegerOverflow=off  InputSameDT=off
  Switch1 : Switch  Criteria=u2 > Threshold  SaturateOnIntegerOverflow=off  InputSameDT=off
  Switch2 : Switch  Criteria=u2 > Threshold  SaturateOnIntegerOverflow=off  InputSameDT=off
  Temperatur unter Rolle : FromWorkspace  VariableName=data_ist_temp_uZR  SampleTime=-1  OutputAfterFinalValue=Setting to zero
  Temperaturen : Scope  NumInputPorts=4
  Transportverzögerung Bandleistung : TransportDelay  DelayTime=12
  Transportverzögerung Heizleistung Betrieb : TransportDelay  DelayTime=93  BufferSize=15000
  Transportverzögerung Heizleistung Stillstand : TransportDelay  DelayTime=150  BufferSize=15000
  Transportverzögerung air knife : TransportDelay  DelayTime=0  BufferSize=20480
  Traverse unten : FromWorkspace  VariableName=data_traverse_down  SampleTime=-1
  Wasserkühlleistung : FromWorkspace  VariableName=data_vzst_kuehl  SampleTime=-1
  Wärmestrom durch Band : Subsystem
  "Wärmeverluste durch Strahlung und Konvektion in Abhängigkeit der Zinntemperatur, mit fester Umgebungstemperatur" : Lookup_n-D  NumberOfTableDimensions=1  BreakpointsForDimension1=[0 250 260 270 280 290 300 310 320]  Table=[0;17000;17200;17400;17600;17800;18000;18200;18400]  InternalRulePriority=Speed  RndMeth=Simplest
  Zinnbadmasse : Constant  Value=7700
  dyn. Bandlänge : FromWorkspace  VariableName=data_bandlaenge  SampleTime=-1
  spez. Wärmekapazität Zinn : Constant  Value=cpSn
  y-Out : Scope  NumInputPorts=2
  wires:
  PID Controller2/1 -> Manual Switch2/1  "Matlab-Regler"
  Manual Switch2/1 -> Gain9/1
  Switch2/1 -> Divide/1
  Gain10/1 -> Switch2/3  "Wirkleistung Stillstand"
  Korrektur Leistung/1 -> Add1/6
  Product1/1 -> PID in Paralellform/3, PID Controller1/4  "D-Anteil Paralellform"
  Divide1/1 -> PID Controller1/3, PID in Paralellform/2  "I-Anteil Parallelform"
  Bandbreite/1 -> Wärmestrom durch Band/4(Bandbreite), Gain6/1, OPC UA Write/8  "Bandbreite in mm"
  1-D Lookup Table2/1 -> OPC UA Write/6, Product1/2  "D-Anteil Zeitdarstellung"
  1-D Lookup Table1/1 -> Divide1/2, OPC UA Write/5  "I-Anteil Zeitdarstellung"
  1-D Lookup Table/1 -> OPC UA Write/4, PID Controller1/2, PID in Paralellform/1, Divide1/1, Product1/1  "P-Anteil"
  Manual Switch1/1 -> Gain4/1, Manual Switch/1
  Gain9/1 -> Manual Switch1/1  "Matlabregler"
  MATLAB Function1/1(korrHeiz) -> ?
  Gain7/1 -> Manual Switch1/2
  Counter Limited/1 -> Scope2/1, OPC UA Write/11
  Constant2/1 -> OPC UA Write/10
  Add1/1 -> Gain3/1, Gain10/1  "Resultierende Leistung"
  Add2/1 -> Alle Leistungen/7  "Summe Verlustleistung"
  OPC UA Read/3 -> Scope1/3
  OPC UA Read/1 -> y-Out/1, Gain7/1, Scope1/1, Display/1  "Siemens-Regler"
  OPC UA Read/2 -> Scope1/2
  Constant1/1 -> Switch1/1
  Add/1 -> Saturation/1
  Gain1/1 -> Add2/1, Alle Leistungen/2, Add/2  "Wasserkühlung"
  Wasserkühlleistung/1 -> Gain1/1  "Wasserkühlleistung in kW"
  Rückschaltung/1 -> Switch1/2
  Switch1/1 -> Add2/5, Alle Leistungen/6, Add1/5  "Traversenleistung"
  Traverse unten/1 -> Gain8/1, Rückschaltung/1
  Transportverzögerung Heizleistung Stillstand/1 -> Switch/3
  Transportverzögerung Heizleistung Betrieb/1 -> Switch/1
  Gain8/1 -> Switch1/3
  Switch/1 -> Alle Leistungen/1, Add1/1  "Heizleistung"
  dyn. Bandlänge/1 -> Scope/1, MATLAB Function1/3(bandlaenge)
  Bandtransport/1 -> MATLAB Function/1(Zustand_Bandlauf), Switch/2, Switch2/2, MATLAB Function1/2(zustand)  "Bandlaufzustand"
  Solltemperautur Stillstand/1 -> MATLAB Function/2(Solltemp_Stillstand), Temperaturen/1  "Solltemperatur Stillstand"
  MATLAB Function/1(y) -> Sum/1, OPC UA Write/1, Sollwert/1  "Sollwert in °C"
  Gain6/1 -> Bandparameter/1  "Bandbreite in m"
  Wärmestrom durch Band/2(Massenstrom für Regler Band) -> 1-D Lookup Table2/1, 1-D Lookup Table1/1, 1-D Lookup Table/1, OPC UA Write/3, Massenstrom/1  "Massenstrom Band für Regler in kg/s"
  Constant/1 -> PID Controller1/5  "N-Filter"
  Wärmestrom durch Band/1(Leistung Band) -> Saturation1/1
  Temperatur unter Rolle/1 -> Temperaturen/4  "Reale Temperatur unter Rolle"
  Gain3/1 -> Switch2/1  "Wirkleistung Betrieb"
  Kühlleistung in Abhängigkeit des Betriebszustand/1 -> Saturation2/1
  "Wärmeverluste durch Strahlung und Konvektion in Abhängigkeit der Zinntemperatur, mit fester Umgebungstemperatur"/1 -> Add1/3, Add2/3, Alle Leistungen/4  "Strahlung und Konvektion in Watt"
  Ofenleistung/1 -> Gain2/1, Gain/1  "Ofenleistung in kW"
  Zinnbadmasse/1 -> Product/2
  AirkniveUS/1 -> Air knife Betriebszustandsberechnung in Prozent/2(druck2)
  Integration/1 -> Temperaturen/3, Sum/2, "Wärmeverluste durch Strahlung und Konvektion in Abhängigkeit der Zinntemperatur, mit fester Umgebungstemperatur"/1, Wärmestrom durch Band/2(Temperatur unter Rolle), OPC UA Write/2  "Simulierte Temp. unter Rolle in °C"
  Sum/1 -> PID Controller1/1, PID Controller2/1
  Gain2/1 -> Heizleistung/2  "Echte Heizleistung"
  Soll-Temp/1 -> Temperaturen/2, MATLAB Function/3(Solltemp_Betrieb)  "Solltemperatur Betrieb"
  Air knife Betriebszustandsberechnung in Prozent/1(Prozent) -> Kühlleistung in Abhängigkeit des Betriebszustand/1
  Manual Switch/1 -> Add/1
  Divide/1 -> Integration/1
  AirkniveOS/1 -> Air knife Betriebszustandsberechnung in Prozent/1(druck1)
  spez. Wärmekapazität Zinn/1 -> Product/1
  Gain4/1 -> Gain5/1
  Gain/1 -> Manual Switch/2
  Bandgeschwindigkeit/1 -> Wärmestrom durch Band/3(Bandgeschwindikeit), Speed/1, OPC UA Write/7  "Bandgeschwindigkeit in m/min"
  Gain5/1 -> Heizleistung/1  "Geregelte simulierte Heizleistung"
  Saturation/1 -> Transportverzögerung Heizleistung Betrieb/1, Transportverzögerung Heizleistung Stillstand/1  "Ofenleistung in Watt"
  Legierung als Nummer/1 -> Legierungsnummer/1, Wärmestrom durch Band/1(Bandnummer)
  Banddicke/1 -> Wärmestrom durch Band/5(Banddicke), Bandparameter/2, OPC UA Write/9  "Banddicke in mm"
  Transportverzögerung Bandleistung/1 -> Add1/2, Add2/2, Alle Leistungen/3  "Bandleistung"
  Saturation2/1 -> Transportverzögerung air knife/1  "Erzwungene Konvektion  durchs air knife in Watt"
  Transportverzögerung air knife/1 -> Add2/4, Alle Leistungen/5, Add1/4  "Air knife Leistung"
  PID Controller1/1 -> y-Out/2, Manual Switch2/2  "Matlab-Regler"
  Saturation1/1 -> Transportverzögerung Bandleistung/1  "Bandleistung in Watt"
  Product/1 -> Divide/2

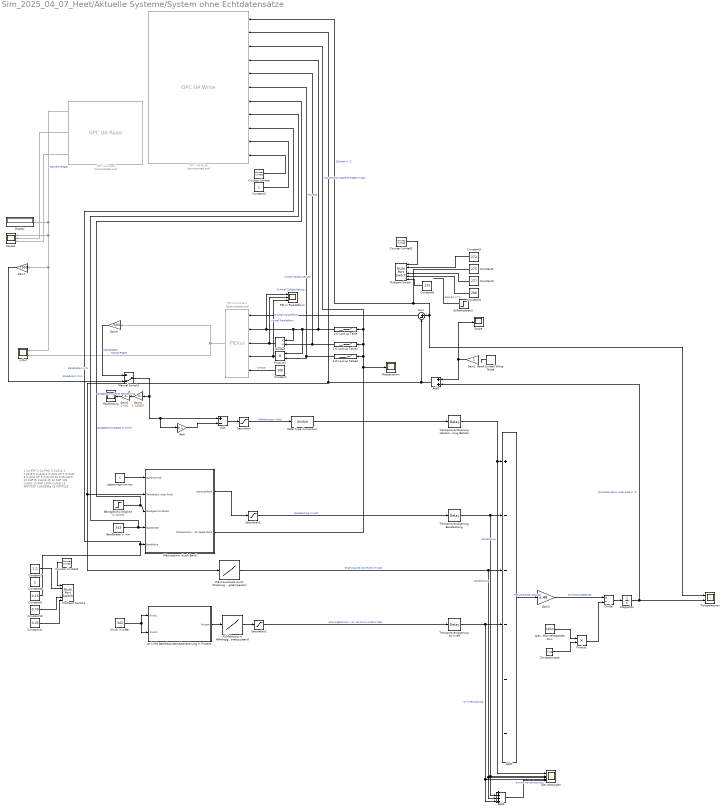
== system Sim_2025_04_07_Heet/Aktuelle Systeme/System ohne Echtdatensätze ==
  note: 1
      | Cu-ETP
      |
      | 2
      | Cu-PHC
      |
      | 3
      | CuSn4
      |
      | 4
      | CuSn5
      |
      | 5
      | CuSn6
      |
      | 6
      | CuSn6 HP
      |
      | 7
      | CuSn8
      |
      | 8
      | CuSn8 HP
      |
      | 9
      | CuSn10
      |
      | 10
      | CuSn3Zn9
      |
      | 11
      | KHP15 CuSn0,15
      |
      | 12
      | KHP 102 CuNiSi
      |
      | 13
      | KHP 102M CuNiSi
      |
      | 14
      | KHP7025 CuNi3SiMg
      |
      | 15
      | KHP7026 CuNi2Si
      |
      | 16
      | KHP105 CuNi1Sn0,5
      |
      | 17
      | KHP109 CuNi1Sn0,9
      |
      | 18
      | C688 CuZn23Al3,5Co
  1-D Lookup Table : Lookup_n-D  NumberOfTableDimensions=1  BreakpointsForDimension1=[0 0.29999999999999999 0.59999999999999998 0.90000000000000002 1.2 1.5 1.8 2.1000000000000001 2.3999999999999999 2.7000000000000002 3 3.2999999999999998 3.6000000000000001 3.8999999999999999 4.2000000000000002 4.5]  Table=[5;5.2;5.4;5.6;5.8;6;6.2;6.4;6.6;6.8;7;7.2;7.4;7.6;7.8;8]  InternalRulePriority=Speed  RndMeth=Simplest
  1-D Lookup Table1 : Lookup_n-D  NumberOfTableDimensions=1  BreakpointsForDimension1=[0 0.29999999999999999 0.59999999999999998 0.90000000000000002 1.2 1.5 1.8 2.1000000000000001 2.3999999999999999 2.7000000000000002 3 3.2999999999999998 3.6000000000000001 3.8999999999999999 4.2000000000000002 4.5]  Table=[250;260;270;280;290;300;310;320;330;340;350;360;370;380;390;400]  InternalRulePriority=Speed  RndMeth=Simplest
  1-D Lookup Table2 : Lookup_n-D  NumberOfTableDimensions=1  BreakpointsForDimension1=[0 0.29999999999999999 0.59999999999999998 0.90000000000000002 1.2 1.5 1.8 2.1000000000000001 2.3999999999999999 2.7000000000000002 3 3.2999999999999998 3.6000000000000001 3.8999999999999999 4.2000000000000002 4.5]  Table=[60;57.7;55.6;53.6;51.7;50;48.4;46.9;45.5;44.1;42.9;41.7;40.5;39.5;38.5;37.5]  InternalRulePriority=Speed  RndMeth=Simplest
  Add : Sum  Inputs=+-
  Add1 : Sum  Inputs=+-----
  Add2 : Sum  Inputs=++++
  Add3 : Sum
  Air knife Betriebszustandsberechnung in Prozent : MATLAB Function  TreatAsAtomicUnit=on  SystemSampleTime=0.1
  Alle Leistungen : Scope  NumInputPorts=6
  Band-Limited White Noise : simulink/Sources/Band-Limited White Noise  Cov=[0.1]  Ts=15  seed=[23341]
  Bandbreite in mm : Constant  Value=343
  Bandgeschwindigkeit in m/min : Step  Time=0  Before=50  After=40  SampleTime=0
  Constant : Constant  Value=100
  Constant1 : Constant  Value=275
  Constant10 : Constant  Value=0.79
  Constant11 : Constant  Value=0.25
  Constant2 : Constant
  Constant3 : Constant  Value=277
  Constant4 : Constant  Value=280
  Constant5 : Constant  Value=272
  Constant6 : Constant  Value=275
  Constant7 : Constant  Value=1.2
  Constant8 : Constant
  Constant9 : Constant  Value=0.15
  Counter Limited : simulink/Sources/Counter Limited  uplimit=100  tsamp=-1
  Counter Limited1 : simulink/Sources/Counter Limited  uplimit=4  tsamp=5000
  Counter Limited2 : simulink/Sources/Counter Limited  uplimit=4  tsamp=3000
  Data Type Conversion : DataTypeConversion  OutDataTypeStr=double  SaturateOnIntegerOverflow=off  RndMeth=Floor
  Display : Display
  Divide : Product  Inputs=*/
  Divide1 : Product  Inputs=*/
  Druck in mBar : Constant  Value=343
  Gain : Gain  Gain=0.1
  Gain1 : Gain
  Gain3 : Gain  Gain=0.48
  Gain4 : Gain  Gain=0.142857
  Gain5 : Gain  Gain=0.001
  Gain7 : Gain  Gain=7000
  Gain9 : Gain  Gain=7000
  Heizleistung : Scope
  Integration : Integrator  InitialCondition=278  IgnoreLimit=on
  Kühlleistung in Abhängigkeit des Betriebszustand : Lookup_n-D  NumberOfTableDimensions=1  BreakpointsForDimension1=[0 50 70 80 90 100]  Table=[0 15000 16500 16700 16900 16800]  InternalRulePriority=Speed  RndMeth=Simplest
  Legierungsnummer : Constant
  Manual Switch1 : ManualSwitch  CurrentSetting=0
  Massenstrom : Scope
  Multiport Switch : MultiPortSwitch  DataPortOrder=Zero-based contiguous  Inputs=5  zeroidx=on  SaturateOnIntegerOverflow=off  InputSameDT=off
  Multiport Switch1 : MultiPortSwitch  DataPortOrder=Zero-based contiguous  Inputs=5  zeroidx=on  SaturateOnIntegerOverflow=off  InputSameDT=off
  OPC UA Read : opcualib/OPC UA Read  Commented=on  SelectedServer=SIMATIC.S7-1500.OPC-UA.Application:PLC_1  ServerList=SIMATIC.S7-1500.OPC-UA.Application:PLC_1  NodeList={ '1', 'reStellwert', '4', '2', '1' }  ShowQualityPort=on  ShowTimestampPort=on  ShowTimestampPortAs=Seconds since start  SampleTime=-1
  OPC UA Write : opcualib/OPC UA Write  Commented=on  SelectedServer=SIMATIC.S7-1500.OPC-UA.Application:PLC_1  ServerList=SIMATIC.S7-1500.OPC-UA.Application:PLC_1  SampleTime=-1  NodeList={ '1', 'reSollwert', '4', '3', '1'; '2', 'reIstTemperaturVonStreckensimulation', '4', '4', '1'; '3', 'reMassenfluss', '4', '5', '1'; '4', 'reP_Anteil', '4', '6', '1'; '5', 'reI_Anteil', '4', '7', '1'; '6', 'reD_Anteil', '4', '8', '1'; '7', 'reGeschwindigkeit', '4', '9', '1'; '8', 'reBandbreite', '4', '10', '1'; '9', 'reBanddicke', '4', '11', '1'; '10', 'boRunVonSimulink', '4', '12', '1'; '11', 'iLifeRegister', '4', '13', '1' }
  PID Controller1 : slpidlib/PID Controller  Commented=on  Controller=PID  Form=Parallel  TimeDomain=Continuous-time  UseExternalTs=off  SampleTime=-1  IntegratorMethod=Forward Euler  FilterMethod=Forward Euler  ControllerParametersSource=external  P=4.4  I=0.02  UseKiTs=off  D=29.92  UseExternalDerivativeSource=off  N=1  UseFilter=on  TunerSelectOption=Transfer Function Based (PID Tuner App)  InitialConditionSource=internal  InitialConditionForIntegrator=0  InitialConditionForFilter=0  DifferentiatorICPrevScaledInput=0  ExternalReset=none  TrackingMode=off  Kt=1  LimitOutput=on  SatLimitsSource=internal  UpperSaturationLimit=100  LowerSaturationLimit=0  LinearizeAsGain=on  AntiWindupMode=none  Kb=1  LimitIntegrator=off  UpperIntegratorSaturationLimit=inf  LowerIntegratorSaturationLimit=-inf  POutMin=[]  POutMax=[]  IOutMin=[]  IOutMax=[]  DOutMin=[]  DOutMax=[]  NOutMin=[]  NOutMax=[]  SumOutMin=[]  SumOutMax=[]  SaturationOutMin=[]  SaturationOutMax=[]  PParamMin=[]  PParamMax=[]  IParamMin=[]  IParamMax=[]  DParamMin=[]  DParamMax=[]  NParamMin=[]  NParamMax=[]  KbParamMin=[]  KbParamMax=[]  KtParamMin=[]  KtParamMax=[]  KbOutMin=[]  KbOutMax=[]  KtOutMin=[]  KtOutMax=[]  IntegratorOutMin=[]  IntegratorOutMax=[]  FilterOutMin=[]  FilterOutMax=[]  SumI1OutMin=[]  SumI1OutMax=[]  SumI2OutMin=[]  SumI2OutMax=[]  SumI3OutMin=[]  SumI3OutMax=[]  SumI4OutMin=[]  SumI4OutMax=[]  SumDOutMin=[]  SumDOutMax=[]  DifferentiatorOutMin=[]  DifferentiatorOutMax=[]  FilterDiffOutCoefMin=[]  FilterDiffOutCoefMax=[]  ReciprocalOutMin=[]  ReciprocalOutMax=[]  SumDenOutMin=[]  SumDenOutMax=[]  SumNumOutMin=[]  SumNumOutMax=[]  DivideOutMin=[]  DivideOutMax=[]  UdiffTsProdOutMin=[]  UdiffTsProdOutMax=[]  NTsProdOutMin=[]  NTsProdOutMax=[]  UintegralTsProdOutMin=[]  UintegralTsProdOutMax=[]  UngainTsProdOutMin=[]  UngainTsProdOutMax=[]  ClampingZeroOutDataTypeStr=Inherit: Inherit via back propagation  ClampingZeroOutMin=[]  ClampingZeroOutMax=[]  FilterDenConstantOutDataTypeStr=Inherit: Inherit via back propagation  FilterDenConstantOutMin=[]  FilterDenConstantOutMax=[]  PCopyOutDataTypeStr=Inherit: Inherit via back propagation  PCopyOutMin=[]  PCopyOutMax=[]  NCopyOutDataTypeStr=Inherit: Inherit via back propagation  NCopyOutMin=[]  NCopyOutMax=[]  IntegratorContinuousStateAttributes=''  IntegratorStateMustResolveToSignalObject=off  IntegratorRTWStateStorageClass=Auto  FilterContinuousStateAttributes=''  FilterStateMustResolveToSignalObject=off  FilterRTWStateStorageClass=Auto  ParallelPVariant=ExternalParameters  IdealPVariant=Disabled  IVariant=ExternalParameters  DVariant=ExternalParameters  IntegratorVariant=Continuous  SatVariant=Enabled  AWVariant=Passthrough  PCopyVariant=Disabled  TRVariant=Disabled  FdbkBlocksVariant=Forward  IdealPFdbkVariant=Disabled  SatFdbkVariant=Disabled  DerivativeFilterVariant=ContFilter  NVariant=ExternalParameters  NCopyVariant=Disabled  FilterICVariant=InternalICsFilter  IntegratorICVariant=InternalICs  ExternalResetVariant=Disabled  TRSumVariant=Passthrough  SumFdbkVariant=Disabled  SumVariant=Sum_PID  TsampFilterVariant=InternalTs  TsampNgainVariant=Passthrough  TsampIntegralVariant=Disabled_SignalSpec  ExternalSaturationOutDataTypeStr=Inherit: Same as second input  DerivativeSourceVariant=ErrorSignal  PreIntVariant=InternalPreInt
  PID in Paralellform : Scope  NumInputPorts=3
  Product : Product
  Product1 : Product
  Saturation : Saturate  UpperLimit=inf  LowerLimit=0
  Saturation1 : Saturate  UpperLimit=inf  LowerLimit=0
  Saturation2 : Saturate  UpperLimit=inf  LowerLimit=0
  Scope : Scope
  Scope1 : Scope  NumInputPorts=3
  Solltemperatur : Step  Time=1000  Before=277  After=279  SampleTime=0
  Sum : Sum  Inputs=|+-
  Temperaturen : Scope  NumInputPorts=2
  Transportverzögerung Bandleistung : TransportDelay  DelayTime=5
  Transportverzögerung Heizleistung Betrieb : TransportDelay  DelayTime=70  BufferSize=15000
  Transportverzögerung air knife : TransportDelay  DelayTime=0  BufferSize=20480
  Wärmestrom durch Band : Subsystem
  "Wärmeverluste durch Strahlung und Konvektion in Abhängigkeit der Zinntemperatur, mit fester Umgebungstemperatur" : Lookup_n-D  NumberOfTableDimensions=1  BreakpointsForDimension1=[0 250 260 270 280 290 300 310 320]  Table=[0;15000;15200;15400;15600;15800;16000;16200;16400]  InternalRulePriority=Speed  RndMeth=Simplest
  Zinnbadmasse : Constant  Value=7700
  spez. Wärmekapazität Zinn : Constant  Value=cpSn
  y-Out : Scope  NumInputPorts=2
  wires:
  Product/1 -> Divide/2
  Saturation1/1 -> Transportverzögerung Bandleistung/1  "Bandleistung in Watt"
  PID Controller1/1 -> y-Out/2, Gain9/1  "Matlab-Regler"
  Transportverzögerung air knife/1 -> Add1/4, Alle Leistungen/5, Add2/4  "Air knife Leistung"
  Saturation2/1 -> Transportverzögerung air knife/1  "Erzwungene Konvektion  durchs air knife in Watt"
  Transportverzögerung Bandleistung/1 -> Alle Leistungen/3, Add2/2, Add1/2  "Bandleistung"
  Constant9/1 -> OPC UA Write/9, Wärmestrom durch Band/5(Banddicke)  "Banddicke in mm"
  Legierungsnummer/1 -> Wärmestrom durch Band/1(Bandnummer)
  Saturation/1 -> Data Type Conversion/1  "Ofenleistung in Watt"
  Gain5/1 -> Heizleistung/1  "Geregelte simulierte Heizleistung"
  Bandgeschwindigkeit in m/min/1 -> OPC UA Write/7, Wärmestrom durch Band/3(Bandgeschwindikeit)  "Bandgeschwindigkeit in m/min"
  Gain4/1 -> Gain5/1
  spez. Wärmekapazität Zinn/1 -> Product/1
  Divide/1 -> Integration/1
  Manual Switch1/1 -> Gain/1, Add/1, Gain4/1
  Air knife Betriebszustandsberechnung in Prozent/1(Prozent) -> Kühlleistung in Abhängigkeit des Betriebszustand/1
  Sum/1 -> PID Controller1/1
  Integration/1 -> Add3/2, Temperaturen/2  "Simulierte Temp. unter Rolle in °C"
  Druck in mBar/1 -> Air knife Betriebszustandsberechnung in Prozent/2(druck2), Air knife Betriebszustandsberechnung in Prozent/1(druck1)
  Zinnbadmasse/1 -> Product/2
  "Wärmeverluste durch Strahlung und Konvektion in Abhängigkeit der Zinntemperatur, mit fester Umgebungstemperatur"/1 -> Alle Leistungen/4, Add2/3, Add1/3  "Strahlung und Konvektion in Watt"
  Kühlleistung in Abhängigkeit des Betriebszustand/1 -> Saturation2/1
  Gain3/1 -> Divide/1  "Wirkleistung Betrieb"
  Wärmestrom durch Band/1(Leistung Band) -> Saturation1/1
  Constant/1 -> PID Controller1/5  "N-Filter"
  Wärmestrom durch Band/2(Massenstrom für Regler Band) -> Massenstrom/1, OPC UA Write/3, 1-D Lookup Table/1, 1-D Lookup Table1/1, 1-D Lookup Table2/1  "Massenstrom Band für Regler in kg/s"
  Constant1/1 -> OPC UA Write/1, Temperaturen/1, Sum/1  "Sollwert in °C"
  Transportverzögerung Heizleistung Betrieb/1 -> Alle Leistungen/1, Add1/1  "Heizleistung"
  Add/1 -> Saturation/1
  OPC UA Read/2 -> Scope1/2
  OPC UA Read/1 -> Display/1, Scope1/1, Gain7/1, y-Out/1  "Siemens-Regler"
  OPC UA Read/3 -> Scope1/3
  Add2/1 -> Alle Leistungen/6  "Summe Verlustleistung"
  Add1/1 -> Gain3/1  "Resultierende Leistung"
  Constant2/1 -> OPC UA Write/10
  Counter Limited/1 -> OPC UA Write/11
  Gain7/1 -> Manual Switch1/2
  Gain9/1 -> Manual Switch1/1  "Matlabregler"
  1-D Lookup Table/1 -> Product1/1, Divide1/1, PID in Paralellform/1, PID Controller1/2, OPC UA Write/4  "P-Anteil"
  1-D Lookup Table1/1 -> OPC UA Write/5, Divide1/2  "I-Anteil Zeitdarstellung"
  1-D Lookup Table2/1 -> Product1/2, OPC UA Write/6  "D-Anteil Zeitdarstellung"
  Bandbreite in mm/1 -> OPC UA Write/8, Wärmestrom durch Band/4(Bandbreite)  "Bandbreite in mm"
  Divide1/1 -> PID in Paralellform/2, PID Controller1/3  "I-Anteil Parallelform"
  Product1/1 -> PID Controller1/4, PID in Paralellform/3  "D-Anteil Paralellform"
  Gain/1 -> Add/2
  Band-Limited White Noise/1 -> ?
  Gain1/1 -> Add3/1, Scope/1
  Data Type Conversion/1 -> Transportverzögerung Heizleistung Betrieb/1
  Solltemperatur/1 -> ?  "Sollwert in °C"
  Constant5/1 -> Multiport Switch/2
  Constant3/1 -> Multiport Switch/4
  Constant4/1 -> Multiport Switch/5
  Counter Limited1/1 -> Multiport Switch/1
  Constant6/1 -> Multiport Switch/6
  Counter Limited2/1 -> Multiport Switch1/1
  Constant7/1 -> Multiport Switch1/2
  ? -> Multiport Switch1/4
  Constant10/1 -> Multiport Switch1/5
  Constant11/1 -> Multiport Switch1/6
  Add3/1 -> OPC UA Write/2, Wärmestrom durch Band/2(Temperatur unter Rolle), "Wärmeverluste durch Strahlung und Konvektion in Abhängigkeit der Zinntemperatur, mit fester Umgebungstemperatur"/1, Sum/2
